simulink model "twr_2017a"  (R2020a)
settings: Solver=FixedStepDiscrete  StartTime=0.0  StopTime=inf  FixedStep=mdl_T_sample  RelTol=1e-3
undefined symbols (not defined in the file or in its folder): ctrl_lqr_addlDyn_A_discrete, ctrl_lqr_addlDyn_B_discrete, ctrl_lqr_addlDyn_C_discrete, ctrl_lqr_addlDyn_D_discrete, ctrl_lqr_addlDyn_k_antiWindup, ctrl_lqr_addlDyn_stateIC, ctrl_lqr_K2, ctrl_motorDriver_v_ff_cmd_v_val, ctrl_motorDriver_v_ff_cmd_v_val_norm_dx_max, ctrl_motorDriver_v_ff_cmd_v_val_norm_dx_min, ctrl_motorDriver_v_output_max, ctrl_motorDriver_v_output_min, ctrl_motorDriver_v_pid_cmd_thetaDot_val, ctrl_motorDriver_v_pid_cmd_thetaDot_val_norm_dx_max, ctrl_motorDriver_v_pid_cmd_thetaDot_val_norm_dx_min, ctrl_motorDriver_v_pid_int_maxVal, ctrl_motorDriver_v_pid_int_minVal, ctrl_motorDriver_v_pid_k_d, ctrl_motorDriver_v_pid_k_i, ctrl_motorDriver_v_pid_k_p, ctrl_motorDriver_v_rts_ss_k_A, ctrl_motorDriver_v_rts_ss_k_B, ctrl_motorDriver_v_rts_ss_k_C, ctrl_motorDriver_v_rts_ss_k_D, ctrl_motorDriver_v_rts_ss_stateIC, ctrl_motorDriver_v_sfr_cmd_p_x_f, ctrl_motorDriver_v_sfr_cmd_p_x_mag, ctrl_motorDriver_v_sfr_cmd_p_y_f, ctrl_motorDriver_v_sfr_cmd_p_y_mag, ctrl_motorDriver_v_sfr_K, ctrl_motorDriver_v_sfr_K_plant, ctrl_motorDriver_v_sfr_K_rts, ctrl_motorDriver_v_T_cmd, ctrl_motorDriver_v_T_init, DiscIntNeverNeededParam, gyro_bias, io_srl_read_rateTransition_initialCondition, k_intmax_uint8, mdl_T_sample, mtr_encoder_filter_z_ss_A, mtr_encoder_filter_z_ss_B, mtr_encoder_filter_z_ss_C, mtr_encoder_filter_z_ss_D, plant, plant_accel_k_digital2analog, plant_body_l_c, plant_body_l_w, plant_gyro_bias_movingAverage_n_pts, plant_gyro_encoder_filter_z_den, plant_gyro_encoder_filter_z_num, plant_gyro_filter_z_den, plant_gyro_filter_z_num, plant_gyro_k_digital2analog, plant_linear_A_continuous, plant_linear_B_continuous, plant_linear_C_continuous, plant_linear_D_continuous, plant_linear_ss_stateIC, plant_linear_ss_t_A, plant_linear_ss_t_B ... (+10)
libraries: svdutilitieslib x135, simulink x57, arduinolib x15, MinSegLibrary_M2V3 x3, dspindex x3, RASPlib x2
(part 3 of 6)

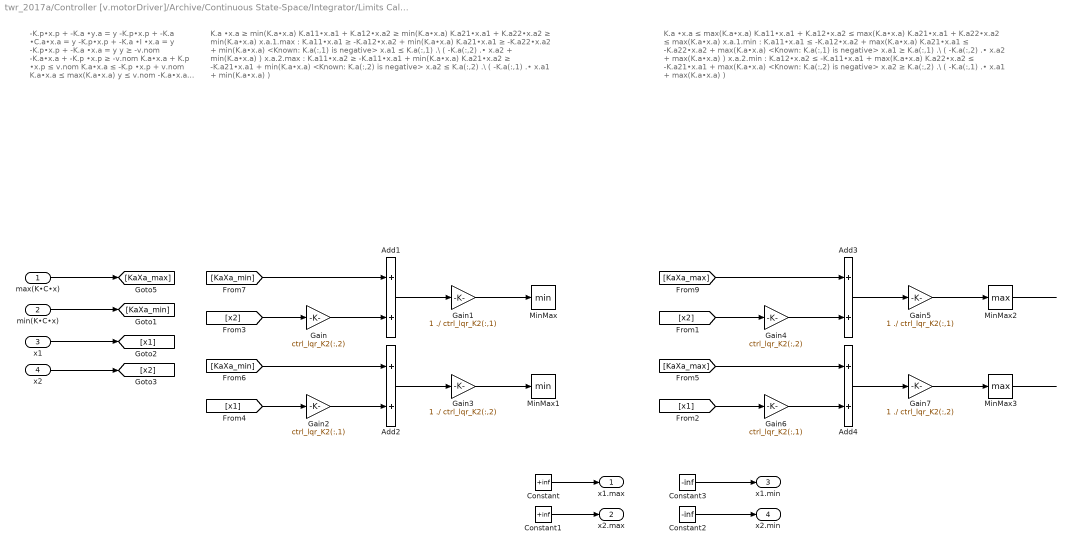
== system twr_2017a/Controller [v.motorDriver]/Archive/Continuous State-Space/Integrator/Limits Calculation ==
  note: K.a •x.a ≥ min(K.a•x.a)
      |
      | K.a11•x.a1 + K.a12•x.a2 ≥ min(K.a•x.a)
      | K.a21•x.a1 + K.a22•x.a2 ≥ min(K.a•x.a)
      |
      | x.a.1.max :
      |
      | K.a11•x.a1 ≥ -K.a12•x.a2 + min(K.a•x.a)
      | K.a21•x.a1 ≥ -K.a22•x.a2 + min(K.a•x.a)
      |
      | <Known: K.a(:,1) is negative>
      |
      | x.a1 ≤ K.a(:,1) .\ ( -K.a(:,2) .• x.a2 + min(K.a•x.a) )
      |
      | x.a.2.max :
      |
      | K.a11•x.a2 ≥ -K.a11•x.a1 + min(K.a•x.a)
      | K.a21•x.a2 ≥ -K.a21•x.a1 + min(K.a•x.a)
      |
      | <Known: K.a(:,2) is negative>
      |
      | x.a2 ≤ K.a(:,2) .\ ( -K.a(:,1) .• x.a1 + min(K.a•x.a) )
  note: K.a •x.a ≤ max(K.a•x.a)
      |
      | K.a11•x.a1 + K.a12•x.a2 ≤ max(K.a•x.a)
      | K.a21•x.a1 + K.a22•x.a2 ≤ max(K.a•x.a)
      |
      | x.a.1.min :
      |
      | K.a11•x.a1 ≤ -K.a12•x.a2 + max(K.a•x.a)
      | K.a21•x.a1 ≤ -K.a22•x.a2 + max(K.a•x.a)
      |
      | <Known: K.a(:,1) is negative>
      |
      | x.a1 ≥ K.a(:,1) .\ ( -K.a(:,2) .• x.a2 + max(K.a•x.a) )
      |
      | x.a.2.min :
      |
      | K.a12•x.a2 ≤ -K.a11•x.a1 + max(K.a•x.a)
      | K.a22•x.a2 ≤ -K.a21•x.a1 + max(K.a•x.a)
      |
      | <Known: K.a(:,2) is negative>
      |
      | x.a2 ≥ K.a(:,2) .\ ( -K.a(:,1) .• x.a1 + max(K.a•x.a) )
  note: -K.p•x.p + -K.a •y.a = y
      | -K.p•x.p + -K.a •C.a•x.a = y
      | -K.p•x.p + -K.a •I •x.a = y
      | -K.p•x.p + -K.a •x.a = y
      |
      | y ≥ -v.nom
      | -K.a•x.a + -K.p •x.p ≥ -v.nom
      | K.a•x.a + K.p •x.p ≤ v.nom
      | K.a•x.a ≤ -K.p •x.p + v.nom
      | K.a•x.a ≤ max(K.a•x.a)
      |
      | y ≤ v.nom
      | -K.a•x.a + -K.p •x.p ≤ v.nom
      | K.a•x.a + K.p •x.p ≥ -v.nom
      | K.a•x.a ≥ -K.p •x.p + -v.nom
      | K.a•x.a ≥ min(K.a•x.a)
  max(K•C•x) : Inport
  min(K•C•x) : Inport  Port=2
  x1 : Inport  Port=3
  x2 : Inport  Port=4
  Add{1..4} (4 alike) : Sum
  Constant : Constant  Value=+inf  SampleTime=mdl_T_sample
  Constant1 : Constant  Value=+inf  SampleTime=mdl_T_sample
  Constant2 : Constant  Value=-inf  SampleTime=mdl_T_sample
  Constant3 : Constant  Value=-inf  SampleTime=mdl_T_sample
  Gain : Gain  Gain=ctrl_lqr_K2(:,2)
      settings: AttributesFormatString=%<Gain>
  Gain1 : Gain  Gain=1 ./ ctrl_lqr_K2(:,1)
      settings: AttributesFormatString=%<Gain>
  Gain2 : Gain  Gain=ctrl_lqr_K2(:,1)
      settings: AttributesFormatString=%<Gain>
  Gain3 : Gain  Gain=1 ./ ctrl_lqr_K2(:,2)
      settings: AttributesFormatString=%<Gain>
  Gain4 : Gain  Gain=ctrl_lqr_K2(:,2)
      settings: AttributesFormatString=%<Gain>
  Gain5 : Gain  Gain=1 ./ ctrl_lqr_K2(:,1)
      settings: AttributesFormatString=%<Gain>
  Gain6 : Gain  Gain=ctrl_lqr_K2(:,1)
      settings: AttributesFormatString=%<Gain>
  Gain7 : Gain  Gain=1 ./ ctrl_lqr_K2(:,2)
      settings: AttributesFormatString=%<Gain>
  MinMax : MinMax
  MinMax1 : MinMax
  MinMax2 : MinMax  Function=max
  MinMax3 : MinMax  Function=max
  x1.max : Outport
  x2.max : Outport  Port=2
  x1.min : Outport  Port=3
  x2.min : Outport  Port=4
  wires:
  Constant/1 -> x1.max/1
  Constant1/1 -> x2.max/1
  Constant3/1 -> x1.min/1
  Constant2/1 -> x2.min/1
  MinMax3/1 -> ?
  MinMax2/1 -> ?
  Gain4/1 -> Add3/2
  [x2] -> Gain4/1
  [KaXa_max] -> Add3/1
  Add3/1 -> Gain5/1
  Gain5/1 -> MinMax2/1
  Gain7/1 -> MinMax3/1
  Add4/1 -> Gain7/1
  [x1] -> Gain6/1
  Gain6/1 -> Add4/2
  [KaXa_max] -> Add4/1
  [KaXa_min] -> Add2/1
  Gain2/1 -> Add2/2
  [x1] -> Gain2/1
  Add2/1 -> Gain3/1
  Gain3/1 -> MinMax1/1
  Gain1/1 -> MinMax/1
  Add1/1 -> Gain1/1
  [KaXa_min] -> Add1/1
  [x2] -> Gain/1
  Gain/1 -> Add1/2
  x2/1 -> [x2]
  x1/1 -> [x1]
  min(K•C•x)/1 -> [KaXa_min]
  max(K•C•x)/1 -> [KaXa_max]

== system twr_2017a/Controller [v.motorDriver]/Archive/Continuous State-Space/Integrator/x1 ==
  u.max : Inport
  u.dot : Inport  Port=2
  u.min : Inport  Port=3
  reset : Inport  Port=4
  Add : Sum  Inputs=-+
  Add1 : Sum
  Constant : Constant  Value=0  SampleTime=mdl_T_sample
  Gain : Gain  Gain=k_antiWindup
      settings: AttributesFormatString=%<Gain>
  Integrator : Integrator  ExternalReset=level hold  InitialCondition=u_init
      settings: AttributesFormatString=initial condition: %<InitialCondition>
  Saturation Dynamic : simulink/Discontinuities/Saturation Dynamic  OutMin=[]  OutMax=[]  OutDataTypeStr=Inherit: Same as second input  OutDataType=fixdt(1, 16)  OutScaling=2^-10  DoSatur=off
  Saturation flag : Subsystem
  x.saturating : MultiPortSwitch  DataPortOrder=Zero-based contiguous  Inputs=2  zeroidx=on
  u : Outport
  x.sat : Outport  Port=2
  wires:
  [u_sat] -> Add/2
  [u_noSat] -> Add/1
  Add1/1 -> x.saturating/2
  Gain/1 -> Add1/2
  Add/1 -> Gain/1
  [x_sat] -> x.saturating/1
  [x_sat] -> x.sat/1
  Saturation flag/1(x.saturating) -> [x_sat]
  [u_noSat] -> Saturation flag/3(u.noSat)
  u.dot/1 -> [u_dot]
  u.max/1 -> [u_max]
  u.min/1 -> [u_min]
  [u_min] -> Saturation flag/4(u.min)
  [u_max] -> Saturation flag/2(u.max)
  [u_dot] -> Saturation flag/1(u.dot)
  [u_dot] -> Add1/1
  [u_sat] -> u/1
  Saturation Dynamic/1 -> [u_sat]
  [u_min] -> Saturation Dynamic/3
  [u_noSat] -> Saturation Dynamic/2
  [u_max] -> Saturation Dynamic/1
  Integrator/1 -> [u_noSat]
  x.saturating/1 -> Integrator/1
  Constant/1 -> x.saturating/3
  reset/1 -> Integrator/2

== system twr_2017a/Controller [v.motorDriver]/Archive/Continuous State-Space/Integrator/x2 ==
  u.max : Inport
  u.dot : Inport  Port=2
  u.min : Inport  Port=3
  reset : Inport  Port=4
  Add : Sum  Inputs=-+
  Add1 : Sum
  Constant : Constant  Value=0  SampleTime=mdl_T_sample
  Gain : Gain  Gain=k_antiWindup
      settings: AttributesFormatString=%<Gain>
  Integrator : Integrator  ExternalReset=level hold  InitialCondition=u_init
      settings: AttributesFormatString=initial condition: %<InitialCondition>
  Saturation Dynamic : simulink/Discontinuities/Saturation Dynamic  OutMin=[]  OutMax=[]  OutDataTypeStr=Inherit: Same as second input  OutDataType=fixdt(1, 16)  OutScaling=2^-10  DoSatur=off
  Saturation flag : Subsystem
  x.saturating : MultiPortSwitch  DataPortOrder=Zero-based contiguous  Inputs=2  zeroidx=on
  u : Outport
  x.sat : Outport  Port=2
  wires:
  reset/1 -> Integrator/2
  Constant/1 -> x.saturating/3
  x.saturating/1 -> Integrator/1
  Integrator/1 -> [u_noSat]
  [u_max] -> Saturation Dynamic/1
  [u_noSat] -> Saturation Dynamic/2
  [u_min] -> Saturation Dynamic/3
  Saturation Dynamic/1 -> [u_sat]
  [u_sat] -> u/1
  [u_dot] -> Add1/1
  [u_dot] -> Saturation flag/1(u.dot)
  [u_max] -> Saturation flag/2(u.max)
  [u_min] -> Saturation flag/4(u.min)
  u.min/1 -> [u_min]
  u.max/1 -> [u_max]
  u.dot/1 -> [u_dot]
  [u_noSat] -> Saturation flag/3(u.noSat)
  Saturation flag/1(x.saturating) -> [x_sat]
  [x_sat] -> x.sat/1
  [x_sat] -> x.saturating/1
  Add/1 -> Gain/1
  Gain/1 -> Add1/2
  Add1/1 -> x.saturating/2
  [u_noSat] -> Add/1
  [u_sat] -> Add/2

== system twr_2017a/Controller [v.motorDriver]/Controller and Enable/Controller/Feed-Forward/Pass-Through ==
  In1 : Inport
  In2 : Inport  Port=2
  Out1 : Outport
  Out2 : Outport  Port=2
  wires:
  In1/1 -> Out1/1
  In2/1 -> Out2/1

== system twr_2017a/Controller [v.motorDriver]/Controller and Enable/Controller/PID/Left-Connected Motor ==
  command : Inport
  measured : Inport  Port=2
  Add : Sum  Inputs=+-
  Add1 : Sum  Inputs=+++
  Derivative : Gain  Gain=ctrl_motorDriver_v_pid_k_d
      settings: AttributesFormatString=%<Gain>
  Discrete Derivative : simulink/Discrete/Discrete Derivative  gainval=1.0  ICPrevScaledInput=0  OutMin=[]  OutMax=[]  OutDataType=fixdt(1, 16)  OutScaling=2^-10  DoSatur=off
      settings: AttributesFormatString=initialCondition = %<ICPrevScaledInput>
  Discrete-Time Integrator : DiscreteIntegrator  SampleTime=-1  LimitOutput=on  UpperSaturationLimit=ctrl_motorDriver_v_pid_int_maxVal  LowerSaturationLimit=ctrl_motorDriver_v_pid_int_minVal  ICPrevOutput=DiscIntNeverNeededParam  ICPrevScaledInput=DiscIntNeverNeededParam
      settings: AttributesFormatString=|
      | initialCondition = %<InitialCondition>
      | maxVal = %<UpperSaturationLimit>
      | minVal = %<LowerSaturationLimit>
  Integration : Gain  Gain=ctrl_motorDriver_v_pid_k_i
      settings: AttributesFormatString=%<Gain>
  Proportional : Gain  Gain=ctrl_motorDriver_v_pid_k_p
      settings: AttributesFormatString=%<Gain>
  output : Outport
  error : Outport  Port=2
  wires:
  Proportional/1 -> Add1/1
  Add/1 -> error/1, Derivative/1, Integration/1, Proportional/1  "error"
  measured/1 -> Add/2
  command/1 -> Add/1
  Integration/1 -> Discrete-Time Integrator/1
  Derivative/1 -> Discrete Derivative/1
  Discrete-Time Integrator/1 -> Add1/2
  Discrete Derivative/1 -> Add1/3
  Add1/1 -> output/1

== system twr_2017a/Controller [v.motorDriver]/Controller and Enable/Controller/PID/Middle-Connected Motor ==
  command : Inport
  measured : Inport  Port=2
  Add : Sum  Inputs=+-
  Add1 : Sum  Inputs=+++
  Derivative : Gain  Gain=ctrl_motorDriver_v_pid_k_d
      settings: AttributesFormatString=%<Gain>
  Discrete Derivative : simulink/Discrete/Discrete Derivative  gainval=1.0  ICPrevScaledInput=0  OutMin=[]  OutMax=[]  OutDataType=fixdt(1, 16)  OutScaling=2^-10  DoSatur=off
      settings: AttributesFormatString=initialCondition = %<ICPrevScaledInput>
  Discrete-Time Integrator : DiscreteIntegrator  SampleTime=-1  LimitOutput=on  UpperSaturationLimit=ctrl_motorDriver_v_pid_int_maxVal  LowerSaturationLimit=ctrl_motorDriver_v_pid_int_minVal  ICPrevOutput=DiscIntNeverNeededParam  ICPrevScaledInput=DiscIntNeverNeededParam
      settings: AttributesFormatString=|
      | initialCondition = %<InitialCondition>
      | maxVal = %<UpperSaturationLimit>
      | minVal = %<LowerSaturationLimit>
  Integration : Gain  Gain=ctrl_motorDriver_v_pid_k_i
      settings: AttributesFormatString=%<Gain>
  Proportional : Gain  Gain=ctrl_motorDriver_v_pid_k_p
      settings: AttributesFormatString=%<Gain>
  output : Outport
  error : Outport  Port=2
  wires:
  Add1/1 -> output/1
  Discrete Derivative/1 -> Add1/3
  Discrete-Time Integrator/1 -> Add1/2
  Derivative/1 -> Discrete Derivative/1
  Integration/1 -> Discrete-Time Integrator/1
  command/1 -> Add/1
  measured/1 -> Add/2
  Add/1 -> Proportional/1, Integration/1, Derivative/1, error/1  "error"
  Proportional/1 -> Add1/1

== system twr_2017a/Controller [v.motorDriver]/Controller and Enable/Controller/State Feedback Regulation/bus2mux [Command] ==
  bus : Inport
  Bus Selector : BusSelector  OutputSignals=theta_global_average [rad],phi_y [rad]
  Constant : Constant  Value=0  SampleTime=mdl_T_sample
  Mux2 : Mux  Inputs=6
  mux : Outport
  wires:
  Bus Selector/2 -> Mux2/5  "<phi_y [rad]>"
  Bus Selector/1 -> Mux2/1  "<theta_global_average [rad]>"
  bus/1 -> Bus Selector/1
  Mux2/1 -> mux/1
  [o] -> Mux2/3, Mux2/4, Mux2/2
  [o] -> Mux2/6
  Constant/1 -> [o]

== system twr_2017a/Controller [v.motorDriver]/Controller and Enable/Controller/State Feedback Regulation/bus2mux [State] ==
  bus : Inport
  Bus Selector1 : BusSelector  OutputSignals=wheel_angularPosition_theta_global_average [rad],body_angularPosition_phi_x [rad],wheel_angularVelocity_thetaDot_global_average [rad/s],body_angularVelocity_phiDot_x [rad/s],body_angularPosition_phi_y [rad],body_angularVelocity_phiDot_y [rad/s]
  Mux1 : Mux  Inputs=6
  mux : Outport
  wires:
  Bus Selector1/1 -> Mux1/1  "<wheel_angularPosition_theta_global_average [rad]>"
  Bus Selector1/6 -> Mux1/6  "<body_angularVelocity_phiDot_y [rad/s]>"
  Bus Selector1/4 -> Mux1/4  "<body_angularVelocity_phiDot_x [rad/s]>"
  Bus Selector1/3 -> Mux1/3  "<wheel_angularVelocity_thetaDot_global_average [rad/s]>"
  Bus Selector1/5 -> Mux1/5  "<body_angularPosition_phi_y [rad]>"
  Bus Selector1/2 -> Mux1/2  "<body_angularPosition_phi_x [rad]>"
  bus/1 -> Bus Selector1/1
  Mux1/1 -> mux/1

== system twr_2017a/Controller [v.motorDriver]/Controller and Enable/Controller/State Feedback Regulation/mux2bus [error] ==
  mux : Inport
  Bus Creator8 : BusCreator  Inputs=6
  Demux1 : Demux  Outputs=6
  bus : Outport
  wires:
  Demux1/6 -> Bus Creator8/6  "phi_y_dot [rad/s]"
  Demux1/2 -> Bus Creator8/2  "phi_x [rad]"
  Demux1/3 -> Bus Creator8/3  "theta_global_average_dot [rad/s]"
  Demux1/4 -> Bus Creator8/4  "phi_x_dot [rad/s]"
  Demux1/5 -> Bus Creator8/5  "phi_y [rad]"
  Demux1/1 -> Bus Creator8/1  "theta_global_average [rad]"
  Bus Creator8/1 -> bus/1
  mux/1 -> Demux1/1

== system twr_2017a/Controller [v.motorDriver]/Controller and Enable/Controller/State Feedback Regulation with Reference Tracking System/bus2mux [Command: Reference Tracking System] ==
  bus : Inport
  Bus Selector : BusSelector  OutputSignals=theta_global_average [rad],phi_y [rad]
  Mux2 : Mux  Inputs=2
  mux : Outport
  wires:
  Mux2/1 -> mux/1
  bus/1 -> Bus Selector/1
  Bus Selector/1 -> Mux2/1  "<theta_global_average [rad]>"
  Bus Selector/2 -> Mux2/2  "<phi_y [rad]>"

== system twr_2017a/Controller [v.motorDriver]/Controller and Enable/Controller/State Feedback Regulation with Reference Tracking System/bus2mux [State: Plant] ==
  bus : Inport
  Bus Selector1 : BusSelector  OutputSignals=wheel_angularPosition_theta_global_average [rad],body_angularPosition_phi_x [rad],wheel_angularVelocity_thetaDot_global_average [rad/s],body_angularVelocity_phiDot_x [rad/s],body_angularPosition_phi_y [rad],body_angularVelocity_phiDot_y [rad/s]
  Mux1 : Mux  Inputs=6
  mux : Outport
  wires:
  Mux1/1 -> mux/1
  bus/1 -> Bus Selector1/1
  Bus Selector1/2 -> Mux1/2  "<body_angularPosition_phi_x [rad]>"
  Bus Selector1/5 -> Mux1/5  "<body_angularPosition_phi_y [rad]>"
  Bus Selector1/3 -> Mux1/3  "<wheel_angularVelocity_thetaDot_global_average [rad/s]>"
  Bus Selector1/4 -> Mux1/4  "<body_angularVelocity_phiDot_x [rad/s]>"
  Bus Selector1/6 -> Mux1/6  "<body_angularVelocity_phiDot_y [rad/s]>"
  Bus Selector1/1 -> Mux1/1  "<wheel_angularPosition_theta_global_average [rad]>"

== system twr_2017a/Controller [v.motorDriver]/Controller and Enable/Controller/State Feedback Regulation with Reference Tracking System/bus2mux [State: Reference Tracking System] ==
  bus : Inport
  Bus Selector2 : BusSelector  OutputSignals=wheel_angularPosition_theta_global_average [rad],body_angularPosition_phi_y [rad]
  Mux : Mux  Inputs=2
  mux : Outport
  wires:
  bus/1 -> Bus Selector2/1
  Bus Selector2/2 -> Mux/2  "<body_angularPosition_phi_y [rad]>"
  Mux/1 -> mux/1
  Bus Selector2/1 -> Mux/1  "<wheel_angularPosition_theta_global_average [rad]>"

== system twr_2017a/Controller [v.motorDriver]/Controller and Enable/Controller/State Feedback Regulation with Reference Tracking System/mux2bus [Error: Reference Tracking System] ==
  mux : Inport
  Bus Creator8 : BusCreator  Inputs=2
  Demux1 : Demux  Outputs=2
  bus : Outport
  wires:
  Bus Creator8/1 -> bus/1
  Demux1/2 -> Bus Creator8/2  "phi_y [rad]"
  Demux1/1 -> Bus Creator8/1  "theta_global_average [rad]"
  mux/1 -> Demux1/1

== system twr_2017a/Plant/Hardware/Analog to Digital Conversion/Motor Driver/Left-Connected ==
  note: Normalize by supply voltage
  voltage.command.analog : Inport
  Abs : Abs
  Compare To Zero : simulink/Logic and Bit Operations/Compare To Zero  relop=<  OutDataTypeStr=boolean
  Constant : Constant  Value=0  SampleTime=mdl_T_sample
  Constant1 : Constant  Value=0  OutDataTypeStr=uint8  SampleTime=mdl_T_sample
  Gain : Gain  Gain=k_intmax_uint8  RndMeth=Round
      settings: AttributesFormatString=%<Gain>
  Gain3 : Gain  Gain=1 / plant_mtr_supply_v
      settings: AttributesFormatString=%<Gain>
  Multiport Switch : MultiPortSwitch  DataPortOrder=Zero-based contiguous  Inputs=2  zeroidx=on
  Multiport Switch1 : MultiPortSwitch  DataPortOrder=Specify indices  Inputs=2  DataPortIndices={1,0}
  Saturation : Saturate  UpperLimit=+1  LowerLimit=-1
  voltage.command.digital.positive : Outport
  voltage.command.digital.negative : Outport  Port=2
  wires:
  Abs/1 -> Gain3/1
  [magnitude] -> Multiport Switch1/2
  [sign] -> Multiport Switch1/1
  Constant1/1 -> Multiport Switch1/3
  Multiport Switch1/1 -> voltage.command.digital.negative/1
  Multiport Switch/1 -> voltage.command.digital.positive/1
  Constant/1 -> Multiport Switch/3
  [sign] -> Multiport Switch/1
  [magnitude] -> Multiport Switch/2
  Gain/1 -> [magnitude]  "|v|.digital"
  Saturation/1 -> Gain/1
  Compare To Zero/1 -> [sign]
  Gain3/1 -> Saturation/1  "|v|.norm"
  voltage.command.analog/1 -> Compare To Zero/1, Abs/1  "v.analog"

== system twr_2017a/Plant/Hardware/Analog to Digital Conversion/Motor Driver/Middle-Connected ==
  note: Normalize by supply voltage
  voltage.command.analog : Inport
  Abs : Abs
  Compare To Zero : simulink/Logic and Bit Operations/Compare To Zero  relop=<  OutDataTypeStr=boolean
  Constant : Constant  Value=0  SampleTime=mdl_T_sample
  Constant1 : Constant  Value=0  OutDataTypeStr=uint8  SampleTime=mdl_T_sample
  Gain : Gain  Gain=k_intmax_uint8  RndMeth=Round
      settings: AttributesFormatString=%<Gain>
  Gain3 : Gain  Gain=1 / plant_mtr_supply_v
      settings: AttributesFormatString=%<Gain>
  Multiport Switch : MultiPortSwitch  DataPortOrder=Zero-based contiguous  Inputs=2  zeroidx=on
  Multiport Switch1 : MultiPortSwitch  DataPortOrder=Specify indices  Inputs=2  DataPortIndices={1,0}
  Saturation : Saturate  UpperLimit=+1  LowerLimit=-1
  voltage.command.digital.positive : Outport
  voltage.command.digital.negative : Outport  Port=2
  wires:
  voltage.command.analog/1 -> Abs/1, Compare To Zero/1  "v.analog"
  Gain3/1 -> Saturation/1  "|v|.norm"
  Compare To Zero/1 -> [sign]
  Saturation/1 -> Gain/1
  Gain/1 -> [magnitude]  "|v|.digital"
  [magnitude] -> Multiport Switch/2
  [sign] -> Multiport Switch/1
  Constant/1 -> Multiport Switch/3
  Multiport Switch/1 -> voltage.command.digital.positive/1
  Multiport Switch1/1 -> voltage.command.digital.negative/1
  Constant1/1 -> Multiport Switch1/3
  [sign] -> Multiport Switch1/1
  [magnitude] -> Multiport Switch1/2
  Abs/1 -> Gain3/1

== system twr_2017a/Plant/Hardware/Arduino Pin IO/Digital Outputs (Writes to Pins)/Motor ==
  motor.left.voltage.command.digital.positive : Inport
  motor.left.voltage.command.digital.negative : Inport  Port=2
  motor.middle.voltage.command.digital.positive : Inport  Port=3
  motor.middle.voltage.command.digital.negative : Inport  Port=4
  Left-Connected : Subsystem
  Right-Connected : Subsystem
  wires:
  motor.left.voltage.command.digital.positive/1 -> Left-Connected/1(motor.left.voltage.command.digital.positive)
  motor.left.voltage.command.digital.negative/1 -> Left-Connected/2(motor.left.voltage.command.digital.negative)
  motor.middle.voltage.command.digital.positive/1 -> Right-Connected/1(motor.middle.voltage.command.digital.positive)
  motor.middle.voltage.command.digital.negative/1 -> Right-Connected/2(motor.middle.voltage.command.digital.negative)

== system twr_2017a/Plant/Hardware/Calculations/Body Angular Position (phi)/X (Pitch) ==
  gyroscope.x : Inport
  accelerometer.y : Inport  Port=2
  accelerometer.z : Inport  Port=3
  clock.timedEvent.plant.x_initialization : Inport  Port=4
  Accelerometer : Subsystem  VariantControl=plant_hardware_calculation_phi_x_accel_var
  Complementary Filter Gyroscope + Accelerometer (Incomplete) : Subsystem  VariantControl=plant_hardware_calculation_phi_x_gyroAndAccel_var
  Gyroscope : Subsystem  VariantControl=(default)
  " position.x" : Outport
  velocity.x : Outport  Port=2

== system twr_2017a/Plant/Hardware/Calculations/Body Angular Position (phi)/Y (Yaw) ==
  gyroscope.y : Inport
  wheel.angularPosition.global.left : Inport  Port=2
  wheel.angularPosition.global.middle : Inport  Port=3
  clock.timedEvent.plant.x_initialization : Inport  Port=4
  Gyroscope : Subsystem  VariantControl=plant_hardware_calculation_phi_y_gyro_var
  Wheel Position : Subsystem  VariantControl=(default)
  " position.y" : Outport
  velocity.y : Outport  Port=2

== system twr_2017a/Plant/Hardware/Calculations/Body Angular Position (phi)/Z (Roll) ==
  gyroscope.z : Inport
  accelerometer.x : Inport  Port=2
  accelerometer.y : Inport  Port=3
  accelerometer.z : Inport  Port=4
  clock.timedEvent.plant.x_initialization : Inport  Port=5
  Accelerometer : Subsystem  VariantControl=plant_hardware_calculation_phi_z_accel_var
  Complementary Filter Gyroscope + Accelerometer (Incomplete) : Subsystem  VariantControl=plant_hardware_calculation_phi_z_gyroAndAccel_var
  Gyroscope : Subsystem  VariantControl=(default)
  position.z : Outport
  velocity.z : Outport  Port=2

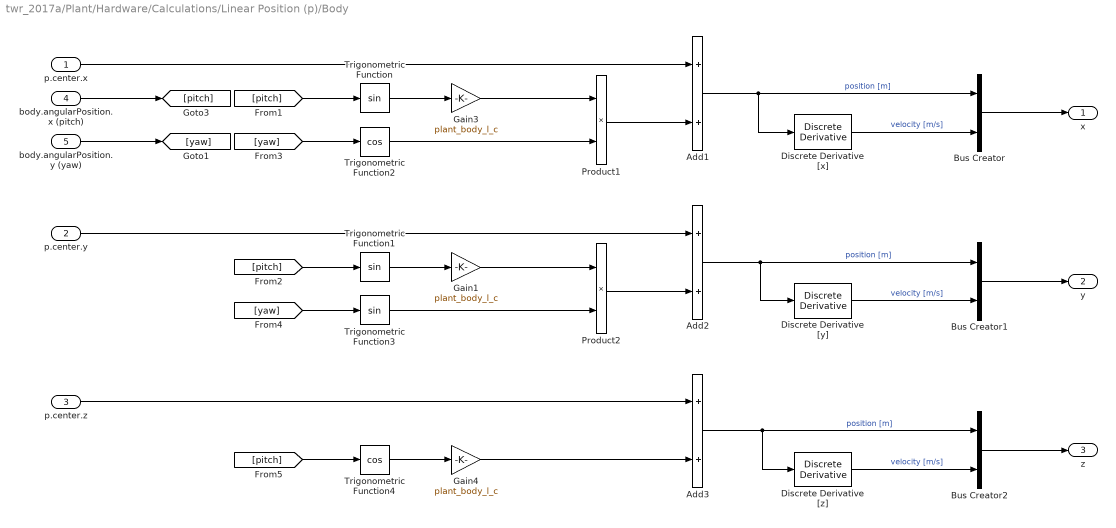
== system twr_2017a/Plant/Hardware/Calculations/Linear Position (p)/Body ==
  p.center.x : Inport
  p.center.y : Inport  Port=2
  p.center.z : Inport  Port=3
  body.angularPosition.x (pitch) : Inport  Port=4
  body.angularPosition.y (yaw) : Inport  Port=5
  Add1 : Sum
  Add2 : Sum
  Add3 : Sum
  Bus Creator : BusCreator  Inputs=2
  Bus Creator1 : BusCreator  Inputs=2
  Bus Creator2 : BusCreator  Inputs=2
  Discrete Derivative [x] : simulink/Discrete/Discrete Derivative  gainval=1.0  ICPrevScaledInput=0  OutMin=[]  OutMax=[]  OutDataType=fixdt(1, 16)  OutScaling=2^-10  DoSatur=off
      settings: AttributesFormatString=initialCondition = %<ICPrevScaledInput>
  Discrete Derivative [y] : simulink/Discrete/Discrete Derivative  gainval=1.0  ICPrevScaledInput=0  OutMin=[]  OutMax=[]  OutDataType=fixdt(1, 16)  OutScaling=2^-10  DoSatur=off
      settings: AttributesFormatString=initialCondition = %<ICPrevScaledInput>
  Discrete Derivative [z] : simulink/Discrete/Discrete Derivative  gainval=1.0  ICPrevScaledInput=0  OutMin=[]  OutMax=[]  OutDataType=fixdt(1, 16)  OutScaling=2^-10  DoSatur=off
      settings: AttributesFormatString=initialCondition = %<ICPrevScaledInput>
  Gain1 : Gain  Gain=plant_body_l_c
      settings: AttributesFormatString=%<Gain>
  Gain3 : Gain  Gain=plant_body_l_c
      settings: AttributesFormatString=%<Gain>
  Gain4 : Gain  Gain=plant_body_l_c
      settings: AttributesFormatString=%<Gain>
  Product1 : Product
  Product2 : Product
  Trigonometric Function : Trigonometry
  Trigonometric Function1 : Trigonometry
  Trigonometric Function2 : Trigonometry  Operator=cos
  Trigonometric Function3 : Trigonometry
  Trigonometric Function4 : Trigonometry  Operator=cos
  x : Outport
  y : Outport  Port=2
  z : Outport  Port=3
  wires:
  Bus Creator1/1 -> y/1
  Discrete Derivative [y]/1 -> Bus Creator1/2  "velocity [m/s]"
  Bus Creator2/1 -> z/1
  Discrete Derivative [z]/1 -> Bus Creator2/2  "velocity [m/s]"
  Add3/1 -> Discrete Derivative [z]/1, Bus Creator2/1  "position [m]"
  Trigonometric Function/1 -> Gain3/1
  Product1/1 -> Add1/2
  Discrete Derivative [x]/1 -> Bus Creator/2  "velocity [m/s]"
  Bus Creator/1 -> x/1
  [pitch] -> Trigonometric Function/1
  Add1/1 -> Discrete Derivative [x]/1, Bus Creator/1  "position [m]"
  body.angularPosition.x (pitch)/1 -> [pitch]
  p.center.x/1 -> Add1/1
  Add2/1 -> Discrete Derivative [y]/1, Bus Creator1/1  "position [m]"
  p.center.y/1 -> Add2/1
  body.angularPosition.y (yaw)/1 -> [yaw]
  Gain3/1 -> Product1/1
  [yaw] -> Trigonometric Function2/1
  Trigonometric Function2/1 -> Product1/2
  Trigonometric Function3/1 -> Product2/2
  [yaw] -> Trigonometric Function3/1
  Gain1/1 -> Product2/1
  [pitch] -> Trigonometric Function1/1
  Product2/1 -> Add2/2
  Trigonometric Function1/1 -> Gain1/1
  [pitch] -> Trigonometric Function4/1
  Gain4/1 -> Add3/2
  Trigonometric Function4/1 -> Gain4/1
  p.center.z/1 -> Add3/1

== system twr_2017a/Plant/Hardware/Calculations/Linear Position (p)/Wheel ==
  wheel.angularVelocity.global : Inport
  body.angularPosition.y (yaw) : Inport  Port=2
  Bus Creator : BusCreator  Inputs=3
  Bus Creator1 : BusCreator  Inputs=3
  Bus Creator2 : BusCreator  Inputs=3
  Bus Selector3 : BusSelector  OutputSignals=x.position [m],y.position [m],z.position [m]
  Bus Selector4 : BusSelector  OutputSignals=x.position [m],y.position [m],z.position [m]
  Center : Subsystem
  Left-Connected : Subsystem
  Middle-Connected : Subsystem
  left : Outport
  middle : Outport  Port=2
  center : Outport  Port=3
  wires:
  Bus Creator/1 -> left/1
  Bus Creator1/1 -> middle/1
  body.angularPosition.y (yaw)/1 -> [yaw]
  wheel.angularVelocity.global/1 -> Center/1(wheel.angularVelocity.global)
  Left-Connected/1(x) -> Bus Creator/1  "x"
  Left-Connected/2(y) -> Bus Creator/2  "y"
  Left-Connected/3(z) -> Bus Creator/3  "z"
  Middle-Connected/1(x) -> Bus Creator1/1  "x"
  Middle-Connected/2(y) -> Bus Creator1/2  "y"
  Middle-Connected/3(z) -> Bus Creator1/3  "z"
  Center/1(x) -> Bus Creator2/1  "x"
  Center/2(y) -> Bus Creator2/2  "y"
  Center/3(z) -> Bus Creator2/3  "z"
  Bus Creator2/1 -> [p_center], center/1
  [yaw] -> Center/2(body.angularPosition.y (yaw))
  [yaw] -> Middle-Connected/4(body.angularPosition.y (yaw))
  [p_center] -> Bus Selector3/1
  Bus Selector3/1 -> Middle-Connected/1(p.center.x)  "<position [m]>"
  Bus Selector3/2 -> Middle-Connected/2(p.center.y)  "<position [m]>"
  Bus Selector3/3 -> Middle-Connected/3(p.center.z)  "<position [m]>"
  Bus Selector4/3 -> Left-Connected/3(p.center.z)  "<position [m]>"
  Bus Selector4/2 -> Left-Connected/2(p.center.y)  "<position [m]>"
  Bus Selector4/1 -> Left-Connected/1(p.center.x)  "<position [m]>"
  [p_center] -> Bus Selector4/1
  [yaw] -> Left-Connected/4(body.angularPosition.y (yaw))

== system twr_2017a/Plant/Hardware/Calculations/Wheel Angular Position (theta)/Reference Point: Body ==
  motorEncoder.left : Inport
  motorEncoder.middle : Inport  Port=2
  Add : Sum
  Bus Creator : BusCreator  Inputs=2
  Bus Creator1 : BusCreator  Inputs=2
  Bus Creator2 : BusCreator  Inputs=2
  Bus Selector1 : BusSelector  OutputSignals=position [rad]
  Bus Selector2 : BusSelector  OutputSignals=position [rad]
  Discrete Derivative [Average] : simulink/Discrete/Discrete Derivative  gainval=1.0  ICPrevScaledInput=0  OutMin=[]  OutMax=[]  OutDataType=fixdt(1, 16)  OutScaling=2^-10  DoSatur=off
      settings: AttributesFormatString=initialCondition = %<ICPrevScaledInput>
  Discrete Derivative [Left-Connected] : simulink/Discrete/Discrete Derivative  gainval=1.0  ICPrevScaledInput=0  OutMin=[]  OutMax=[]  OutDataType=fixdt(1, 16)  OutScaling=2^-10  DoSatur=off
      settings: AttributesFormatString=initialCondition = %<ICPrevScaledInput>
  Discrete Derivative [Middle-Connected] : simulink/Discrete/Discrete Derivative  gainval=1.0  ICPrevScaledInput=0  OutMin=[]  OutMax=[]  OutDataType=fixdt(1, 16)  OutScaling=2^-10  DoSatur=off
      settings: AttributesFormatString=initialCondition = %<ICPrevScaledInput>
  Discrete Filter: Bessel LPF [Left-Connected] : DiscreteFilter  Numerator=plant_mtr_encoder_filter_z_num  Denominator=plant_mtr_encoder_filter_z_den  SampleTime=mdl_T_sample
      settings: AttributesFormatString=|
      | Num: %<Numerator>
      | Den: %<Denominator>
  Discrete Filter: Bessel LPF [Middle-Connected] : DiscreteFilter  Numerator=plant_mtr_encoder_filter_z_num  Denominator=plant_mtr_encoder_filter_z_den  SampleTime=mdl_T_sample
      settings: AttributesFormatString=|
      | Num: %<Numerator>
      | Den: %<Denominator>
  Gain : Gain  Gain=1/2
  left : Outport
  middle : Outport  Port=2
  average : Outport  Port=3
  wires:
  motorEncoder.left/1 -> Discrete Derivative [Left-Connected]/1, Bus Creator/1  "position [rad]"
  motorEncoder.middle/1 -> Discrete Derivative [Middle-Connected]/1, Bus Creator1/1  "position [rad]"
  Bus Creator2/1 -> average/1
  Gain/1 -> Discrete Derivative [Average]/1, Bus Creator2/1  "position [rad]"
  [middle] -> Bus Selector2/1
  [left] -> Bus Selector1/1
  Bus Creator/1 -> [left], left/1
  Bus Creator1/1 -> [middle], middle/1
  Bus Selector1/1 -> Add/1  "<position [rad]>"
  Bus Selector2/1 -> Add/2  "<position [rad]>"
  Discrete Filter: Bessel LPF [Left-Connected]/1 -> Bus Creator/2  "velocity [rad/s]"
  Discrete Derivative [Middle-Connected]/1 -> Discrete Filter: Bessel LPF [Middle-Connected]/1
  Add/1 -> Gain/1
  Discrete Derivative [Left-Connected]/1 -> Discrete Filter: Bessel LPF [Left-Connected]/1
  Discrete Filter: Bessel LPF [Middle-Connected]/1 -> Bus Creator1/2  "velocity [rad/s]"
  Discrete Derivative [Average]/1 -> Bus Creator2/2  "velocity [rad/s]"

== system twr_2017a/Plant/Hardware/Calculations/Wheel Angular Position (theta)/Reference Point: Earth ==
  wheel.left.angularPosition.body : Inport
  wheel.middle.angularPosition.body : Inport  Port=2
  body.angularPosition.x (pitch) : Inport  Port=3
  Add : Sum
  Add1 : Sum
  Add2 : Sum
  Bus Creator2 : BusCreator  Inputs=2
  Bus Creator4 : BusCreator  Inputs=2
  Bus Creator5 : BusCreator  Inputs=2
  Bus Selector3 : BusSelector  OutputSignals=position [rad]
  Bus Selector4 : BusSelector  OutputSignals=position [rad]
  Discrete Derivative [Average] : simulink/Discrete/Discrete Derivative  gainval=1.0  ICPrevScaledInput=0  OutMin=[]  OutMax=[]  OutDataType=fixdt(1, 16)  OutScaling=2^-10  DoSatur=off
      settings: AttributesFormatString=initialCondition = %<ICPrevScaledInput>
  Discrete Derivative [Left-Connected] : simulink/Discrete/Discrete Derivative  gainval=1.0  ICPrevScaledInput=0  OutMin=[]  OutMax=[]  OutDataType=fixdt(1, 16)  OutScaling=2^-10  DoSatur=off
      settings: AttributesFormatString=initialCondition = %<ICPrevScaledInput>
  Discrete Derivative [Middle-Connected] : simulink/Discrete/Discrete Derivative  gainval=1.0  ICPrevScaledInput=0  OutMin=[]  OutMax=[]  OutDataType=fixdt(1, 16)  OutScaling=2^-10  DoSatur=off
      settings: AttributesFormatString=initialCondition = %<ICPrevScaledInput>
  Gain : Gain  Gain=1/2
  left : Outport
  middle : Outport  Port=2
  average : Outport  Port=3
  wires:
  Bus Creator5/1 -> average/1
  Gain/1 -> Discrete Derivative [Average]/1, Bus Creator5/1  "position [rad]"
  Add1/1 -> Discrete Derivative [Left-Connected]/1, Bus Creator2/1  "position [rad]"
  [left] -> Bus Selector3/1
  Bus Selector4/1 -> Add/2  "<position [rad]>"
  Add/1 -> Gain/1
  Discrete Derivative [Left-Connected]/1 -> Bus Creator2/2  "velocity [rad/s]"
  Bus Selector3/1 -> Add/1  "<position [rad]>"
  Bus Creator4/1 -> [middle], middle/1
  Discrete Derivative [Average]/1 -> Bus Creator5/2  "velocity [rad/s]"
  Add2/1 -> Discrete Derivative [Middle-Connected]/1, Bus Creator4/1  "position [rad]"
  Bus Creator2/1 -> [left], left/1
  [middle] -> Bus Selector4/1
  Discrete Derivative [Middle-Connected]/1 -> Bus Creator4/2  "velocity [rad/s]"
  body.angularPosition.x (pitch)/1 -> [pitch]
  [pitch] -> Add1/2
  wheel.left.angularPosition.body/1 -> Add1/1
  wheel.middle.angularPosition.body/1 -> Add2/1
  [pitch] -> Add2/2

== system twr_2017a/Plant/Hardware/Digital to Analog Conversion/Gyroscope/x ==
  digital : Inport
  clock.timedEvent.plant.x_initialization : Inport  Port=2
  Add : Sum  Inputs=+-
  Constant : Constant  Commented=on  Value=gyro_bias  SampleTime=mdl_T_sample
  Data Type Conversion1 : DataTypeConversion  OutDataTypeStr=double
  Gain : Gain  Gain=plant_gyro_k_digital2analog
      settings: AttributesFormatString=%<Gain>
  Moving Average : Subsystem  mask{N=plant_gyro_bias_movingAverage_n_pts}
      mask prompts: N "Number of samples averaged"
      settings: AttributesFormatString=%<N>
  analog : Outport
  wires:
  Add/1 -> Gain/1
  digital/1 -> Data Type Conversion1/1
  Data Type Conversion1/1 -> Add/1, Moving Average/1(u)
  Gain/1 -> analog/1
  clock.timedEvent.plant.x_initialization/1 -> Moving Average/Enable
  Moving Average/1(u.avg) -> Add/2

== system twr_2017a/Plant/Hardware/Digital to Analog Conversion/Gyroscope/y ==
  digital : Inport
  clock.timedEvent.model.initialization : Inport  Port=2
  Add : Sum  Inputs=+-
  Constant : Constant  Commented=on  Value=gyro_bias  SampleTime=mdl_T_sample
  Data Type Conversion1 : DataTypeConversion  OutDataTypeStr=double
  Gain : Gain  Gain=plant_gyro_k_digital2analog
      settings: AttributesFormatString=%<Gain>
  Moving Average : Subsystem  mask{N=plant_gyro_bias_movingAverage_n_pts}
      mask prompts: N "Number of samples averaged"
      settings: AttributesFormatString=%<N>
  analog : Outport
  wires:
  Moving Average/1(u.avg) -> Add/2
  clock.timedEvent.model.initialization/1 -> Moving Average/Enable
  Gain/1 -> analog/1
  Data Type Conversion1/1 -> Moving Average/1(u), Add/1
  digital/1 -> Data Type Conversion1/1
  Add/1 -> Gain/1

== system twr_2017a/Plant/Hardware/Digital to Analog Conversion/Gyroscope/z ==
  digital : Inport
  clock.timedEvent.model.initialization : Inport  Port=2
  Add : Sum  Inputs=+-
  Constant : Constant  Commented=on  Value=gyro_bias  SampleTime=mdl_T_sample
  Data Type Conversion1 : DataTypeConversion  OutDataTypeStr=double
  Gain : Gain  Gain=plant_gyro_k_digital2analog
      settings: AttributesFormatString=%<Gain>
  Moving Average : Subsystem  mask{N=plant_gyro_bias_movingAverage_n_pts}
      mask prompts: N "Number of samples averaged"
      settings: AttributesFormatString=%<N>
  analog : Outport
  wires:
  Add/1 -> Gain/1
  digital/1 -> Data Type Conversion1/1
  Data Type Conversion1/1 -> Moving Average/1(u), Add/1
  Gain/1 -> analog/1
  clock.timedEvent.model.initialization/1 -> Moving Average/Enable
  Moving Average/1(u.avg) -> Add/2

== system twr_2017a/Plant/Hardware-Equivalent Linear Dynamics/Calculation/Linear Position (p)/Body ==
  p.center.x : Inport
  p.center.y : Inport  Port=2
  p.center.z : Inport  Port=3
  body.angularPosition.x (pitch) : Inport  Port=4
  body.angularPosition.y (yaw) : Inport  Port=5
  Add1 : Sum
  Add2 : Sum
  Add3 : Sum
  Bus Creator : BusCreator  Inputs=2
  Bus Creator1 : BusCreator  Inputs=2
  Bus Creator2 : BusCreator  Inputs=2
  Discrete Derivative (Average) : simulink/Discrete/Discrete Derivative  gainval=1.0  ICPrevScaledInput=0  OutMin=[]  OutMax=[]  OutDataType=fixdt(1, 16)  OutScaling=2^-10  DoSatur=off
      settings: AttributesFormatString=initialCondition = %<ICPrevScaledInput>
  Discrete Derivative (Left-Connected) : simulink/Discrete/Discrete Derivative  gainval=1.0  ICPrevScaledInput=0  OutMin=[]  OutMax=[]  OutDataType=fixdt(1, 16)  OutScaling=2^-10  DoSatur=off
      settings: AttributesFormatString=initialCondition = %<ICPrevScaledInput>
  Discrete Derivative (Middle-Connected) : simulink/Discrete/Discrete Derivative  gainval=1.0  ICPrevScaledInput=0  OutMin=[]  OutMax=[]  OutDataType=fixdt(1, 16)  OutScaling=2^-10  DoSatur=off
      settings: AttributesFormatString=initialCondition = %<ICPrevScaledInput>
  Gain1 : Gain  Gain=plant_body_l_c
      settings: AttributesFormatString=%<Gain>
  Gain3 : Gain  Gain=plant_body_l_c
      settings: AttributesFormatString=%<Gain>
  Gain4 : Gain  Gain=plant_body_l_c
      settings: AttributesFormatString=%<Gain>
  Product1 : Product
  Product2 : Product
  Trigonometric Function : Trigonometry
  Trigonometric Function1 : Trigonometry
  Trigonometric Function2 : Trigonometry  Operator=cos
  Trigonometric Function3 : Trigonometry
  Trigonometric Function4 : Trigonometry  Operator=cos
  x : Outport
  y : Outport  Port=2
  z : Outport  Port=3
  wires:
  Bus Creator1/1 -> y/1
  Discrete Derivative (Middle-Connected)/1 -> Bus Creator1/2  "velocity [m/s]"
  Bus Creator2/1 -> z/1
  Discrete Derivative (Average)/1 -> Bus Creator2/2  "velocity [m/s]"
  Add3/1 -> Discrete Derivative (Average)/1, Bus Creator2/1  "position [m]"
  Trigonometric Function/1 -> Gain3/1
  Product1/1 -> Add1/2
  Discrete Derivative (Left-Connected)/1 -> Bus Creator/2  "velocity [m/s]"
  Bus Creator/1 -> x/1
  [pitch] -> Trigonometric Function/1
  Add1/1 -> Discrete Derivative (Left-Connected)/1, Bus Creator/1  "position [m]"
  body.angularPosition.x (pitch)/1 -> [pitch]
  p.center.x/1 -> Add1/1
  Add2/1 -> Discrete Derivative (Middle-Connected)/1, Bus Creator1/1  "position [m]"
  p.center.y/1 -> Add2/1
  body.angularPosition.y (yaw)/1 -> [yaw]
  Gain3/1 -> Product1/1
  [yaw] -> Trigonometric Function2/1
  Trigonometric Function2/1 -> Product1/2
  Trigonometric Function3/1 -> Product2/2
  [yaw] -> Trigonometric Function3/1
  Gain1/1 -> Product2/1
  [pitch] -> Trigonometric Function1/1
  Product2/1 -> Add2/2
  Trigonometric Function1/1 -> Gain1/1
  [pitch] -> Trigonometric Function4/1
  Gain4/1 -> Add3/2
  Trigonometric Function4/1 -> Gain4/1
  p.center.z/1 -> Add3/1

== system twr_2017a/Plant/Hardware-Equivalent Linear Dynamics/Calculation/Linear Position (p)/Wheel ==
  wheel.angularVelocity.global : Inport
  body.angularPosition.y (yaw) : Inport  Port=2
  Bus Creator : BusCreator  Inputs=3
  Bus Creator1 : BusCreator  Inputs=3
  Bus Creator2 : BusCreator  Inputs=3
  Bus Selector3 : BusSelector  OutputSignals=x.position [m],y.position [m],z.position [m]
  Bus Selector4 : BusSelector  OutputSignals=x.position [m],y.position [m],z.position [m]
  Center : Subsystem
  Left-Connected : Subsystem
  Middle-Connected : Subsystem
  left : Outport
  middle : Outport  Port=2
  center : Outport  Port=3
  wires:
  Bus Creator/1 -> left/1
  Bus Creator1/1 -> middle/1
  body.angularPosition.y (yaw)/1 -> [yaw]
  wheel.angularVelocity.global/1 -> Center/1(wheel.angularVelocity.global)
  Left-Connected/1(x) -> Bus Creator/1  "x"
  Left-Connected/2(y) -> Bus Creator/2  "y"
  Left-Connected/3(z) -> Bus Creator/3  "z"
  Middle-Connected/1(x) -> Bus Creator1/1  "x"
  Middle-Connected/2(y) -> Bus Creator1/2  "y"
  Middle-Connected/3(z) -> Bus Creator1/3  "z"
  Center/1(x) -> Bus Creator2/1  "x"
  Center/2(y) -> Bus Creator2/2  "y"
  Center/3(z) -> Bus Creator2/3  "z"
  Bus Creator2/1 -> [p_center], center/1
  [yaw] -> Center/2(body.angularPosition.y (yaw))
  [yaw] -> Middle-Connected/4(body.angularPosition.y (yaw))
  [p_center] -> Bus Selector3/1
  Bus Selector3/1 -> Middle-Connected/1(p.center.x)  "<position [m]>"
  Bus Selector3/2 -> Middle-Connected/2(p.center.y)  "<position [m]>"
  Bus Selector3/3 -> Middle-Connected/3(p.center.z)  "<position [m]>"
  Bus Selector4/3 -> Left-Connected/3(p.center.z)  "<position [m]>"
  Bus Selector4/2 -> Left-Connected/2(p.center.y)  "<position [m]>"
  Bus Selector4/1 -> Left-Connected/1(p.center.x)  "<position [m]>"
  [p_center] -> Bus Selector4/1
  [yaw] -> Left-Connected/4(body.angularPosition.y (yaw))

== system twr_2017a/Plant/Hardware-Equivalent Linear Dynamics/Calculation/Wheel Angular Position (theta)/Reference Point: Body ==
  wheel.angularPosition.global.left : Inport
  wheel.angularPosition.global.middle : Inport  Port=2
  body.angularPosition.x (pitch) : Inport  Port=3
  Add1 : Sum  Inputs=+-
  Add2 : Sum  Inputs=+-
  Add3 : Sum
  Bus Creator : BusCreator  Inputs=2
  Bus Creator1 : BusCreator  Inputs=2
  Bus Creator2 : BusCreator  Inputs=2
  Bus Selector3 : BusSelector  OutputSignals=position [rad]
  Bus Selector4 : BusSelector  OutputSignals=position [rad]
  Discrete Derivative (Average) : simulink/Discrete/Discrete Derivative  gainval=1.0  ICPrevScaledInput=0  OutMin=[]  OutMax=[]  OutDataType=fixdt(1, 16)  OutScaling=2^-10  DoSatur=off
      settings: AttributesFormatString=initialCondition = %<ICPrevScaledInput>
  Discrete Derivative (Left-Connected) : simulink/Discrete/Discrete Derivative  gainval=1.0  ICPrevScaledInput=0  OutMin=[]  OutMax=[]  OutDataType=fixdt(1, 16)  OutScaling=2^-10  DoSatur=off
      settings: AttributesFormatString=initialCondition = %<ICPrevScaledInput>
  Discrete Derivative (Middle-Connected) : simulink/Discrete/Discrete Derivative  gainval=1.0  ICPrevScaledInput=0  OutMin=[]  OutMax=[]  OutDataType=fixdt(1, 16)  OutScaling=2^-10  DoSatur=off
      settings: AttributesFormatString=initialCondition = %<ICPrevScaledInput>
  Gain : Gain  Gain=1/2
  left : Outport
  middle : Outport  Port=2
  average : Outport  Port=3
  wires:
  Add1/1 -> Discrete Derivative (Left-Connected)/1, Bus Creator/1  "position [rad]"
  Add2/1 -> Discrete Derivative (Middle-Connected)/1, Bus Creator1/1  "position [rad]"
  Discrete Derivative (Left-Connected)/1 -> Bus Creator/2  "velocity [rad/s]"
  Discrete Derivative (Middle-Connected)/1 -> Bus Creator1/2  "velocity [rad/s]"
  [pitch] -> Add1/2
  body.angularPosition.x (pitch)/1 -> [pitch]
  [pitch] -> Add2/2
  Bus Creator2/1 -> average/1
  Discrete Derivative (Average)/1 -> Bus Creator2/2  "velocity [rad/s]"
  Add3/1 -> Gain/1  "position  [rad]"
  Gain/1 -> Discrete Derivative (Average)/1, Bus Creator2/1  "position [rad]"
  Bus Creator1/1 -> [middle], middle/1
  Bus Creator/1 -> [left], left/1
  [middle] -> Bus Selector4/1
  [left] -> Bus Selector3/1
  Bus Selector3/1 -> Add3/1  "<position [rad]>"
  Bus Selector4/1 -> Add3/2  "<position [rad]>"
  wheel.angularPosition.global.left/1 -> Add1/1  "position  [rad]"
  wheel.angularPosition.global.middle/1 -> Add2/1  "velocity  [rad/s]"

== system twr_2017a/Plant/Hardware-Equivalent Linear Dynamics/Calculation/Wheel Angular Position (theta)/Reference Point: Earth ==
  wheel.angularPosition.global.average : Inport
  wheel.angularVelocity.global.average : Inport  Port=2
  body.angularPosition.y (yaw) : Inport  Port=3
  Add1 : Sum  Inputs=+-
  Add2 : Sum
  Bus Creator : BusCreator  Inputs=2
  Bus Creator1 : BusCreator  Inputs=2
  Bus Creator2 : BusCreator  Inputs=2
  Bus Selector1 : BusSelector  OutputSignals=position [rad]
  Bus Selector2 : BusSelector  OutputSignals=position [rad]
  Bus Selector3 : BusSelector  OutputSignals=position [rad]
  Discrete Derivative (Left-Connected) : simulink/Discrete/Discrete Derivative  gainval=1.0  ICPrevScaledInput=0  OutMin=[]  OutMax=[]  OutDataType=fixdt(1, 16)  OutScaling=2^-10  DoSatur=off
      settings: AttributesFormatString=initialCondition = %<ICPrevScaledInput>
  Discrete Derivative (Middle-Connected) : simulink/Discrete/Discrete Derivative  gainval=1.0  ICPrevScaledInput=0  OutMin=[]  OutMax=[]  OutDataType=fixdt(1, 16)  OutScaling=2^-10  DoSatur=off
      settings: AttributesFormatString=initialCondition = %<ICPrevScaledInput>
  Gain : Gain  Gain=plant.body.l.w / (2 * plant.wheel.r)
      settings: AttributesFormatString=%<Gain>
  Gain1 : Gain  Gain=2
  left : Outport
  middle : Outport  Port=2
  average : Outport  Port=3
  wires:
  Discrete Derivative (Left-Connected)/1 -> Bus Creator/2  "velocity [rad/s]"
  Bus Creator2/1 -> [average], average/1
  wheel.angularPosition.global.average/1 -> Bus Creator2/1  "position [rad]"
  Discrete Derivative (Middle-Connected)/1 -> Bus Creator1/2  "velocity [rad/s]"
  Bus Creator/1 -> left/1
  Add1/1 -> Discrete Derivative (Left-Connected)/1, Bus Creator/1  "position [rad]"
  Add2/1 -> Discrete Derivative (Middle-Connected)/1, Bus Creator1/1  "position [rad]"
  [average] -> Bus Selector1/1
  wheel.angularVelocity.global.average/1 -> Bus Creator2/2  "velocity [rad/s]"
  Bus Selector1/1 -> Gain1/1  "<position [rad]>"
  Bus Selector2/1 -> Add2/1  "<position [rad]>"
  [average] -> Bus Selector2/1
  body.angularPosition.y (yaw)/1 -> Gain/1
  Gain/1 -> Add2/2
  Bus Creator1/1 -> [middle], middle/1
  Gain1/1 -> Add1/1
  Bus Selector3/1 -> Add1/2  "<position [rad]>"
  [middle] -> Bus Selector3/1

== system twr_2017a/User IO/Reads (From PC)/Controller/State Feedback Regulation/[x,y] to [magnitude, angle]: p ==
  x : Inport
  y : Inport  Port=2
  Angle : Subsystem
  Magnitude : Subsystem
  magnitude : Outport
  angle : Outport  Port=2
  wires:
  x/1 -> [x]
  y/1 -> [y]
  [x] -> Magnitude/1(u.x)
  [y] -> Magnitude/2(u.y)
  [y] -> Angle/2(u.y)
  [x] -> Angle/1(u.x)
  Magnitude/1(| u |) -> magnitude/1
  Angle/1("< u  ") -> angle/1

== system twr_2017a/User IO/Reads (From PC)/Controller/State Feedback Regulation/[x,y] to [magnitude, angle]: p.dot ==
  x : Inport
  y : Inport  Port=2
  Angle : Subsystem
  Magnitude : Subsystem
  magnitude : Outport
  angle : Outport  Port=2
  wires:
  Angle/1("< u  ") -> angle/1
  Magnitude/1(| u |) -> magnitude/1
  [x] -> Angle/1(u.x)
  [y] -> Angle/2(u.y)
  [y] -> Magnitude/2(u.y)
  [x] -> Magnitude/1(u.x)
  y/1 -> [y]
  x/1 -> [x]

== system twr_2017a/User IO/Reads (From PC)/Controller/State Feedback Regulation/phi.y.discontinuous to phi.y.continuous ==
  note: reduce any change in phi to
      | magnitude less than pi/2
      | by removing a factor of pi.
      |
      | if k is odd, sign change of theta.dot is necessary.
  theta.dot.in : Inport
  phi.y.in : Inport  Port=2
  Add : Sum  Inputs=+-
  Add1 : Sum  Inputs=+-
  Constant1 : Constant  Value=-1  SampleTime=mdl_T_sample
  Gain : Gain  Gain=1 / pi
      settings: AttributesFormatString=%<Gain>
  Gain1 : Gain  Gain=pi
      settings: AttributesFormatString=%<Gain>
  Math Function : Math  Operator=pow  SignedPower=on  SaturateOnIntegerOverflow=on
  Product : Product
  Rounding Function : Rounding  Operator=round
  Unit Delay : UnitDelay  SampleTime=-1  HasFrameUpgradeWarning=on
  theta.dot : Outport
  phi.y : Outport  Port=2
  wires:
  phi.y.in/1 -> Add1/1, Add/1
  theta.dot.in/1 -> Product/1
  Add1/1 -> Gain/1
  Gain/1 -> Rounding Function/1
  Gain1/1 -> Add/2
  Rounding Function/1 -> [n_pi]
  [n_pi] -> Gain1/1
  Constant1/1 -> Math Function/1
  [n_pi] -> Math Function/2
  Math Function/1 -> Product/2
  Product/1 -> theta.dot/1
  Add/1 -> [phi]
  [phi] -> phi.y/1
  [phi] -> Unit Delay/1
  Unit Delay/1 -> Add1/2
